simulink model "blockDiagramTask6"  (R2025a)
settings: Solver=VariableStepAuto  StartTime=0.0  StopTime=3.6  RelTol=1e-3
InitFcn:
  | run motor_specs.m
model workspace: external: MATLAB File motor_specs.m (data not in the file)
values from neighbouring files (symbols this model uses):
  A6 = [ 0, 0, 1, 0 ... (first row only)    [ssAndTF.m]
  B6 = [0, 0, K_M/(J_gm*R), 0]'    [ssAndTF.m]
  b_m = C_V / rpm_to_rs    (= 1.05042262441e-05)    [motor_specs.m]
  C6 = eye(4)    [ssAndTF.m]
  J = 6.3E-6    (= 6.3e-06)    [motor_specs.m]
  K_E = 0.006741 / rpm_to_rs    (= 0.0643718082829)    [motor_specs.m]
  K_M = 0.0644    [motor_specs.m]
  R = 3.23    [motor_specs.m]
  U_N = 36    [motor_specs.m]
libraries: fl_lib x4, nesl_utility x3, ee_lib x1
settings Model: Creator=josef  LastModifiedBy=josef

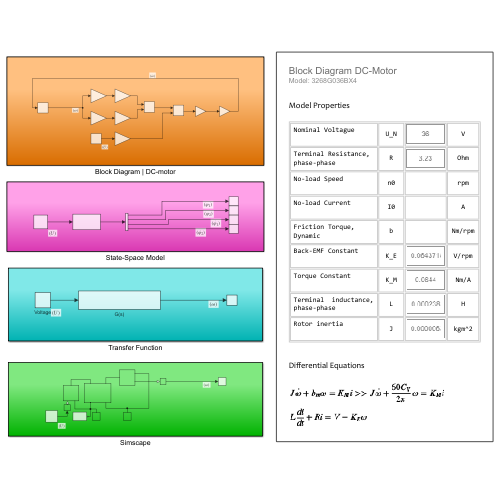
[thumbnail: Simulink's stored preview of the top-level diagram]
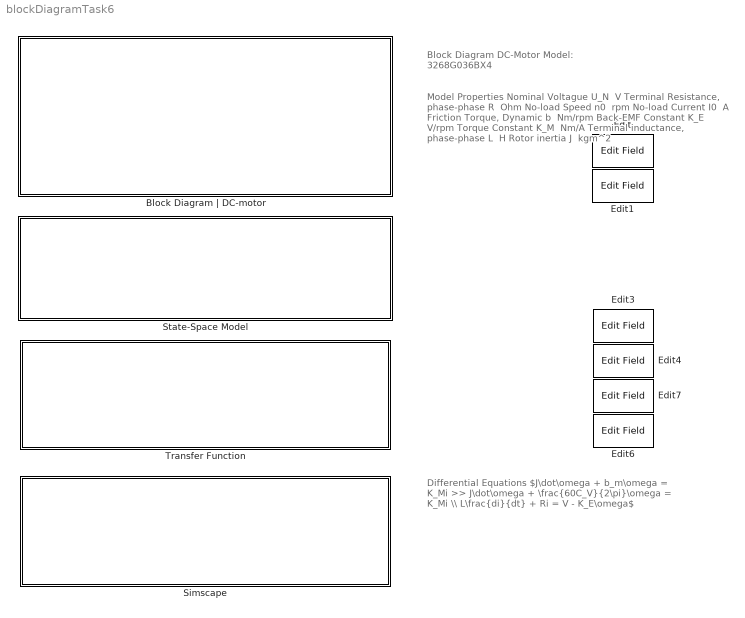
== system blockDiagramTask6 ==
  note: Differential Equations
      |
      | $J\dot\omega + b_m\omega = K_Mi >> J\dot\omega + \frac{60C_V}{2\pi}\omega = K_Mi \\ L\frac{di}{dt} + Ri = V - K_E\omega$
  note: Model Properties
      |
      | Nominal Voltague
      |
      | U_N
      | ​
      | V
      |
      | Terminal Resistance,
      | phase-phase
      | R
      | ​
      | Ohm
      |
      | No-load Speed
      |
      | n0
      | ​
      | rpm
      |
      | No-load Current
      |
      | I0
      | ​
      | A
      |
      | Friction Torque,
      | Dynamic
      | b
      | ​
      | Nm/rpm
      |
      | Back-EMF Constant
      |
      | K_E
      | ​
      | V/rpm
      |
      | Torque Constant
      |
      | K_M
      | ​
      | Nm/A
      |
      | Terminal inductance,
      | phase-phase
      | L
      | ​
      | H
      |
      | Rotor inertia
      |
      | J
      | ​
      | kgm^2
  note: Block Diagram DC-Motor
      | Model: 3268G036BX4
  Block Diagram | DC-motor : Subsystem
  Edit{,1,3..4,6..7} (6 alike) : EditField  LabelPosition=Hide  ShowInitialText=on  Alignment=Center  Opacity=0
  Simscape : Subsystem
  State-Space Model : Subsystem
  Transfer Function : Subsystem

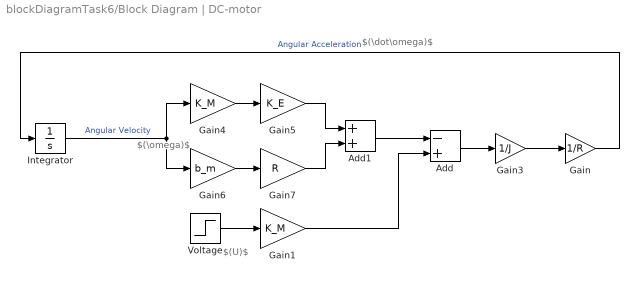
== system blockDiagramTask6/Block Diagram | DC-motor ==
  note: $(\omega)$
  note: $(\dot\omega)$
  note: $(U)$
  Add : Sum  Inputs=-+
  Add1 : Sum
  Gain : Gain  Gain=1/R
  Gain1 : Gain  Gain=K_M
  Gain3 : Gain  Gain=1/J
  Gain4 : Gain  Gain=K_M
  Gain5 : Gain  Gain=K_E
  Gain6 : Gain  Gain=b_m
  Gain7 : Gain  Gain=R
  Integrator : Integrator
  Voltage : Step  Time=0  After=U_N  SampleTime=0
  wires:
  Add1/1 -> Add/1
  Gain4/1 -> Gain5/1
  Gain1/1 -> Add/2
  Gain3/1 -> Gain/1
  Gain5/1 -> Add1/1
  Integrator/1 -> Gain6/1, Gain4/1  "Angular Velocity"
  Gain6/1 -> Gain7/1
  Voltage/1 -> Gain1/1
  Gain/1 -> Integrator/1  "Angular Acceleration"
  Gain7/1 -> Add1/2
  Add/1 -> Gain3/1

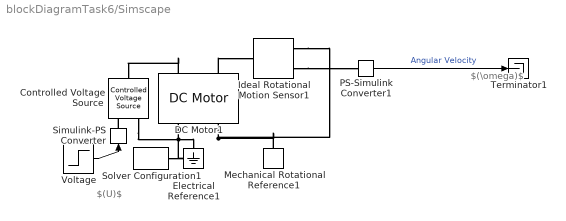
== system blockDiagramTask6/Simscape ==
  note: $(\omega)$
  note: $(U)$
  Controlled Voltage Source : fl_lib/Electrical/Electrical Sources/Controlled Voltage Source
  DC Motor1 : ee_lib/Electromechanical/Brushed Motors/DC Motor  field_option=ee.enum.field_option.pm  Rf=100 Ohm  Lf=1 H  Laf=0.15 H  If0=0 A  parameterization=ee.enum.dcparam_option.circuit_param  Ra=R Ohm  La=0 H  emf_or_torque=ee.enum.emf_or_torque.kv  Kv=K_E V*s/rad  Ki=6.876e-4 N*m/A  T_stall=0.24e-3 N*m  w_max=19100 rpm  w_rated=15000 rpm  P_rated=0.08 W  V_rated=1.5 V  lam_param=ee.enum.lam_param.damping  i_noload=0 A  V_i_noload=1.5 V  J=J kg*m^2  lam=b_m N*m*s/rad  speed0=0 rpm  alpha=3.93e-3 1/K  Tmeas=25 degC  thermal_mass=100 J/K  initial_temperature=25 degC
  Electrical Reference1 : fl_lib/Electrical/Electrical Elements/Electrical Reference
  Ideal Rotational Motion Sensor1 : fl_lib/Mechanical/Mechanical Sensors/Ideal Rotational Motion Sensor  reference=foundation.enum.MeasurementReference.difference  acceleration_port=false  velocity_port=true  position_port=false  wrap_angle=false  offset=0 rad
      settings: InternalSimscapePortConfiguration="{\"Bottom\":[],\"Left\":[{\"id\":\"R\",\"label\":\"R\",\"type\":\"foundation.mechanical.rotational.rotational\"}],\"Right\":[{\"id\":\"C\",\"label\":\"C\",\"type\":\"foundation.mechanical.rotational.rotational\"},{\"id\":\"W\",\"label\":\"W\",\"type\":\"output\"}],\"Top\":[]}"
  Mechanical Rotational Reference1 : fl_lib/Mechanical/Rotational Elements/Mechanical Rotational Reference
  PS-Simulink Converter1 : nesl_utility/PS-Simulink Converter  PhysicalDomain=network_engine_domain  SubClassName=ps_output  LeftPortType=input  RightPortType=output  PseudoPeriodic=off  Frequencies=[]  VectorFormat=inherit  Unit=inherit  AffineConversion=off
  Simulink-PS Converter : nesl_utility/Simulink-PS Converter  PhysicalDomain=network_engine_domain  SubClassName=ps_input  LeftPortType=input  RightPortType=output  PseudoPeriodic=off  Frequencies=[]  NoiseDistribution=none  NoiseParameters=[]  Unit=1  AffineConversion=off  FilteringAndDerivatives=provide  SimscapeFilterOrder=1  InputFilterTimeConstant=0.001  UdotUserProvided=0
  Solver Configuration1 : nesl_utility/Solver Configuration  PhysicalDomain=network_engine_domain  SubClassName=solver  LeftPortType=input  RightPortType=generic  Tones=[]  Harmonics=[]  SimulateNoise=off  Profile=off  UseLocalSampling=off  EnableSwitchedLinearOptims=on  FrequencyDomain=off  UseCCode=off  RelTol=0.001  AbsTol=0.001  MinStep=1e-09  ToWorkspace=off  RevertToSquareIcSolve=off  NumHomotopyIterations=100  PhasorMode=off  PhasorModeNumHarmonics=1  ConsistencySolver=NEWTON_XTOL_AFTER_FTOL  IndexReductionMethod=DerivativeReplacement  DoDC=off  ResidualTolerance=1e-09  ConsistencyTolSource=GLOBAL  ConsistencyAbsTol=0.001  ConsistencyRelTol=0.001  ConsistencyTolFactor=0.001  UseLocalSolver=off  LocalSolverChoice=NE_BACKWARD_EULER_ADVANCER  ResolveIndetEquations=on  FunctionEvalNumThread=1  LocalSolverSampleTime=0.001  DoFixedCost=off  MaxNonlinIter=3  MaxModeIter=2  ComputeImpulses=off  ImpulseIterations=2  LinearAlgebra=auto  LinearAlgebraNumThread=0  EquationFormulation=NE_TIME_EF  DelaysMemoryBudget=1024  AutomaticFiltering=on  FilteringTimeConstant=0.001  PartitionStorageMethod=AS_NEEDED  PartitionMemoryBudget=1024  PartitionMethod=ROBUST  MultibodyUseLocalSolver=off  MultibodyLocalSolverChoice=ODE1  MultibodyLocalSolverSampleTime=0.001
  Terminator1 : Terminator
  Voltage : Step  Time=0.1  After=U_N  SampleTime=0
  wires:
  PS-Simulink Converter1/1 -> Terminator1/1  "Angular Velocity"
  Voltage/1 -> Simulink-PS Converter/1
  connections:
  Solver Configuration1/RConn1 -- Controlled Voltage Source/RConn2 -- Electrical Reference1/LConn1 -- DC Motor1/RConn1
  DC Motor1/RConn2 -- Ideal Rotational Motion Sensor1/RConn1 -- Mechanical Rotational Reference1/LConn1
  Ideal Rotational Motion Sensor1/RConn2 -- PS-Simulink Converter1/LConn1
  Simulink-PS Converter/RConn1 -- Controlled Voltage Source/RConn1
  DC Motor1/LConn1 -- Controlled Voltage Source/LConn1
  DC Motor1/LConn2 -- Ideal Rotational Motion Sensor1/LConn1

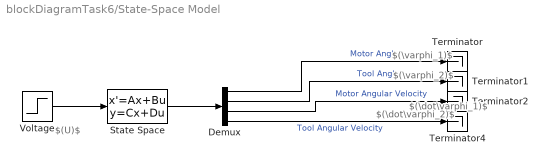
== system blockDiagramTask6/State-Space Model ==
  note: $(\dot\varphi_2)$
  note: $(U)$
  note: $(\dot\varphi_1)$
  note: $(\varphi_2)$
  note: $(\varphi_1)$
  Demux : Demux
  State Space : StateSpace  A=A6  B=B6  C=C6  D=[0;0;0;0]  InitialCondition=0
  Terminator{,1..2,4} (4 alike) : Terminator
  Voltage : Step  Time=0.1  After=U_N  SampleTime=0
  wires:
  Demux/2 -> Terminator1/1  "Tool Angle"
  Demux/4 -> Terminator4/1  "Tool Angular Velocity"
  Demux/1 -> Terminator/1  "Motor Angle"
  Demux/3 -> Terminator2/1  "Motor Angular Velocity"
  State Space/1 -> Demux/1
  Voltage/1 -> State Space/1

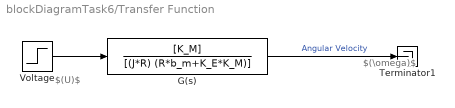
== system blockDiagramTask6/Transfer Function ==
  note: $(\omega)$
  note: $(U)$
  G(s) : TransferFcn  Numerator=[K_M]  Denominator=[(J*R) (R*b_m+K_E*K_M)]
  Terminator1 : Terminator
  Voltage : Step  Time=0.1  After=U_N  SampleTime=0
  wires:
  G(s)/1 -> Terminator1/1  "Angular Velocity"
  Voltage/1 -> G(s)/1
